simulink model "DependableKalmanFilter"  (R2023b)
settings: Solver=VariableStepAuto  StartTime=0.0  StopTime=10.0  RelTol=1e-3
undefined symbols (not defined in the file): gray, Rec, SDTV
libraries: visiontextngfix x2, visionanalysis x2, visionstatistics x1, visionconversions x1, dspvision x1
settings Model: PacingRate=0.011000  Creator=Shiqi  LastModifiedBy=Shiqi

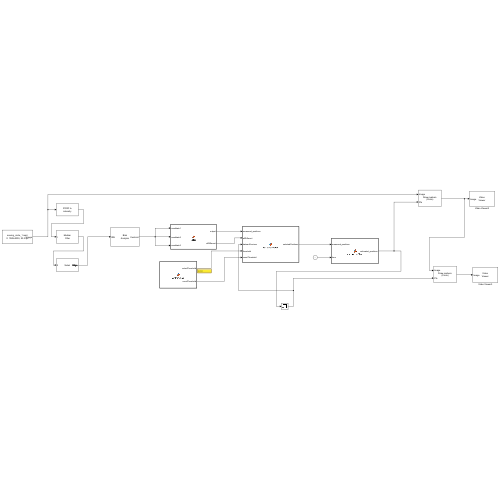
[thumbnail: Simulink's stored preview of the top-level diagram]
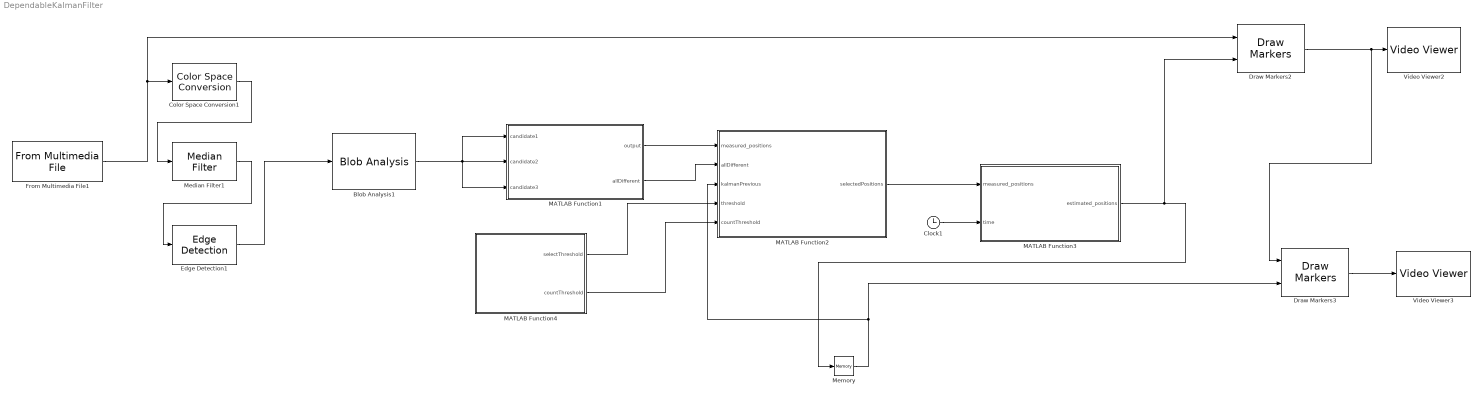
== system DependableKalmanFilter ==
  Blob Analysis1 : visionstatistics/Blob Analysis  Tag=vipblks_row_conv  area=off  centroid=on  bBox=off  majorAxis=off  minorAxis=off  angle=off  eccentricity=off  equivDiameterSq=off  extent=off  perimeter=off  outDT=single  conn=8  isLabel=off  maxBlobs=5  warnIfNumBlobsExceeded=on  isCount=off  useMinArea=off  minArea=0  useMaxArea=off  maxArea=intmax('uint32')  excludeBorderBlob=off  isOutVarDim=off  isFill=on  fillValues=-1  roundingMode=Floor  overflowMode=off  prodOutputMode=Binary point scaling  prodOutputWordLength=32  prodOutputFracLength=16  accumMode=Binary point scaling  accumWordLength=32  accumFracLength=0  outputMode=Binary point scaling  outputWordLength=32  outputFracLength=16  firstCoeffMode=Binary point scaling  firstCoeffWordLength=16  firstCoeffFracLength=14  secondCoeffMode=Binary point scaling  secondCoeffWordLength=32  secondCoeffFracLength=16
  Clock1 : Clock
  Color Space Conversion1 : visionconversions/Color Space  Conversion  conversion=Obsolete  conversionActive=R'G'B' to intensity  wp_str=D65  rec=Rec. 601 (SDTV)  sys=1125/60/2:1  imagePorts=One multidimensional signal
  Draw Markers2 : visiontextngfix/Draw Markers  shape=Circle  size=10  fill=on  fillClrSource=Specify via dialog  display=User-specified value  intensity=200  color=[0 255 0]  opacity=0.6  viewport=Entire image  antialiasing=off  inType=Obsolete  imagePorts=One multidimensional signal  roundingMode=Floor  overflowMode=off  memoryMode=Specify word length  memoryWordLength=16  memoryFracLength=15  prodOutputMode=Binary point scaling  prodOutputWordLength=32  prodOutputFracLength=14
  Draw Markers3 : visiontextngfix/Draw Markers  shape=Circle  size=10  fill=on  fillClrSource=Specify via dialog  display=User-specified value  intensity=200  color=[255 0 0]  opacity=0.6  viewport=Entire image  antialiasing=off  inType=Obsolete  imagePorts=One multidimensional signal  roundingMode=Floor  overflowMode=off  memoryMode=Specify word length  memoryWordLength=16  memoryFracLength=15  prodOutputMode=Binary point scaling  prodOutputWordLength=32  prodOutputFracLength=14
  Edge Detection1 : visionanalysis/Edge Detection  method=Sobel  outputType=Binary image  userDefinedThreshold=off  thresholdSource=Input port  threshold=20  thresholdTuning=4  edgeThinning=off  threshold_canny=[0.25 0.60]  autoPercent=70  sigma=1  roundingMode=Floor  overflowMode=off  prodOutputMode=Binary point scaling  prodOutputWordLength=32  prodOutputFracLength=8
  From Multimedia File1 : dspvision/From Multimedia File  inputFilename=D:\University of Pittsburgh\Courses\ECE2390_Image_Processing_And_Computer_Vision\Assignments\ECE2165_Video_Making\moving_circle_1.mp4  readRange=[1 Inf]  loop=on  numPlays=inf  outputStreams=Video only  videoDataType=double  audioDataType=int16  inheritSampleTime=on  userDefinedSampleTime=1/30  noAudioOutput=off  isIntensityVideo=off  fourcc=RGB  colorVideoFormat=One multidimensional signal  outputEOF=off  dataOrg=Column-major  audioFrameSize=1024  computeAudioFrameSize=off  outSamplingMode=Sample based
      settings: LibrarySourceBlock=visionsources/From Multimedia File
  MATLAB Function1 : MATLAB Function  TreatAsAtomicUnit=on
  MATLAB Function2 : MATLAB Function  TreatAsAtomicUnit=on
  MATLAB Function3 : MATLAB Function  TreatAsAtomicUnit=on
  MATLAB Function4 : MATLAB Function  TreatAsAtomicUnit=on
  Median Filter1 : visionanalysis/Median Filter  nghbood=[3 3]  outSize=Same as input port I  padType=Constant  padSrc=Specify via dialog  padVal=0  roundingMode=Floor  overflowMode=off
  Memory : Memory
  Video Viewer2 : VideoViewer  colormapValue=gray(256)  FigPos=[359.666666666667 1318.66666666667 1143.33333333333 642.666666666667]
  Video Viewer3 : VideoViewer  colormapValue=gray(256)  FigPos=[380.333333333333 959.333333333333 1124 700]
  wires:
  MATLAB Function1/2(allDifferent) -> MATLAB Function2/2(allDifferent)
  MATLAB Function3/1(estimated_positions) -> Draw Markers2/2, Memory/1
  MATLAB Function2/1(selectedPositions) -> MATLAB Function3/1(measured_positions)
  Clock1/1 -> MATLAB Function3/2(time)
  Median Filter1/1 -> Edge Detection1/1
  Color Space Conversion1/1 -> Median Filter1/1
  Edge Detection1/1 -> Blob Analysis1/1
  MATLAB Function1/1(output) -> MATLAB Function2/1(measured_positions)
  Draw Markers2/1 -> Draw Markers3/1, Video Viewer2/1
  Draw Markers3/1 -> Video Viewer3/1
  MATLAB Function4/1(selectThreshold) -> MATLAB Function2/4(threshold)
  MATLAB Function4/2(countThreshold) -> MATLAB Function2/5(countThreshold)
  Blob Analysis1/1 -> MATLAB Function1/3(candidate3), MATLAB Function1/2(candidate2), MATLAB Function1/1(candidate1)
  Memory/1 -> Draw Markers3/2, MATLAB Function2/3(kalmanPrevious)
  From Multimedia File1/1 -> Draw Markers2/1, Color Space Conversion1/1

== matlab function DependableKalmanFilter/MATLAB Function1 ==
  data: candidate1 input; output output; candidate2 input; candidate3 input; allDifferent output
function [output, allDifferent] = voter(candidate1, candidate2, candidate3)
    % Suppose input are M*2 matrix
    % initialize output
    [numBlobs, ~] = size(candidate1); % get nums of blobs
    output = zeros(numBlobs, 2); % init output matrix
    allDifferent = true(numBlobs, 1); % init alldifferent flag to 1
    threshold = 10; % set threshold

    for i = 1:numBlobs
        % compare the position of candidates
        if all(abs(candidate1(i,:) - candidate2(i,:)) < threshold)
            output(i,:) = mean([candidate1(i,:); candidate2(i,:)], 1);
            allDifferent(i) = false; % not all are different
        elseif all(abs(candidate1(i,:) - candidate3(i,:)) < threshold)
            output(i,:) = mean([candidate1(i,:); candidate3(i,:)], 1);
            allDifferent(i) = false;
        elseif all(abs(candidate2(i,:) - candidate3(i,:)) < threshold)
            output(i,:) = mean([candidate2(i,:); candidate3(i,:)], 1);
            allDifferent(i) = false;
        else
            % if all different, use candidate 1
            output(i,:) = candidate1(i,:);
        end
    end
end

== matlab function DependableKalmanFilter/MATLAB Function2 ==
  data: measured_positions input; selectedPositions output; allDifferent input; kalmanPrevious input; threshold input; countThreshold input
function selectedPositions = selectEstimates(measured_positions, allDifferent, kalmanPrevious, threshold, countThreshold)
    persistent deviationCount;
    persistent initCount; % save different count
    [num_objects, ~] = size(measured_positions); % get nums of blobs
    
    % init
    if isempty(deviationCount)
        deviationCount = zeros(num_objects, 1);
    end

    if isempty(initCount)
        initCount = 0;
    end
    
    selectedPositions = zeros(num_objects, 2); % init estimate position

    if(initCount ~= 0)
        initCount = initCount + 1
        for obj_idx = 1:num_objects
            % if alldifferent is true, use kalmanPrevious
            if allDifferent(obj_idx)
                selectedPositions(obj_idx, :) = kalmanPrevious(obj_idx, :);
                deviationCount(obj_idx) = 0; % reset deviationCount
            else
                % calculate how current measured positions differs to
                % kalman previous result
                deviation = abs(measured_positions(obj_idx, :) - kalmanPrevious(obj_idx, :));
    
                % if differences are huge
                if any(deviation > threshold)
                    deviationCount(obj_idx) = deviationCount(obj_idx) + 1; % increase the counter
                    if deviationCount(obj_idx) >= countThreshold
                        % counter greater maximum, accept current
                        % measurement
                        selectedPositions(obj_idx, :) = measured_positions(obj_idx, :);
                        deviationCount(obj_idx) = 0; % reset the counter
                    else
                        % otherwise, keep using kalmanPrevious value
                        selectedPositions(obj_idx, :) = kalmanPrevious(obj_idx, :);
                    end
                else
                    % if not exceed threshold, keep using measured
                    % positions
                    selectedPositions(obj_idx, :) = measured_positions(obj_idx, :);
                    deviationCount(obj_idx) = 0; % reset the counter
                end
            end
        end
    else
        selectedPositions = measured_positions;
    end
    selectedPositions = measured_positions;
    
end

== matlab function DependableKalmanFilter/MATLAB Function3 ==
  data: measured_positions input; estimated_positions output; time input
function estimated_positions = myKalmanFilter(measured_positions, time)
    % Input: 
    % measured_positions: Nx2 matrix, each row is an object's measured x and y position
    % Output: 
    % estimated_positions: Nx2 matrix, each row is an object's estimated x and y position
    
    persistent x_hat P_hat prev_time

    [num_objects, num_dimensions] = size(measured_positions);
    
    % Initialize if persistent variable is null or out of size
    if isempty(x_hat) || isempty(P_hat)
        x_hat = zeros(num_objects, 4); %  Initial estimation
        P_hat = repmat(eye(4), [1 1 num_objects]); %  Initial covariance
    end

    if isempty(prev_time)
        prev_time = 0
    end
    
    delta_t = time - prev_time

    prev_time = time

    A = [1 0 delta_t 0; 0 1 0 delta_t; 0 0 1 0; 0 0 0 1]; %  State transfer matrix

    H = [1 0 0 0; 0 1 0 0]; %  Observation matrix

    Q = 0.2 * eye(4); %  Process noise covariance
    R = 0.0001 * eye(2); %  Measurement noise covariance
    
     
    estimated_positions = zeros(num_objects, num_dimensions); %  Initialization Output
    
    %  Kalman filter for each object
    for obj_idx = 1:num_objects
        %  Extract state estimate and covariance for that object
        x_hat_obj = x_hat(obj_idx, :).';
        P_hat_obj = P_hat(:, :, obj_idx);
        
        %  Prediction
        x_pred = A * x_hat_obj;
        P_pred = A * P_hat_obj * A' + Q;
        
        %  Update
        K = P_pred * H' / (H * P_pred * H' + R);
        x_hat_new = x_pred + K * (measured_positions(obj_idx, :).' - H * x_pred);
        P_hat_new = P_pred - K * H * P_pred;
        
        %  Store the new estimate
        x_hat(obj_idx, :) = x_hat_new.';
        P_hat(:, :, obj_idx) = P_hat_new;
        
        %  Store the estimated position
        estimated_positions(obj_idx, :) = x_hat_new(1:2).';
    end
end

== matlab function DependableKalmanFilter/MATLAB Function4 ==
  data: selectThreshold output; countThreshold output
function [selectThreshold, countThreshold] = setThreshold()
    selectThreshold = 100;
    countThreshold = 5;
